simulink subsystem "s3EM"  (R2023b)
settings: Solver=VariableStepAuto  StartTime=0.0  StopTime=10.0  RelTol=1e-3
settings Model: Creator=The MathWorks, Inc.  LastModifiedBy=The MathWorks, Inc.

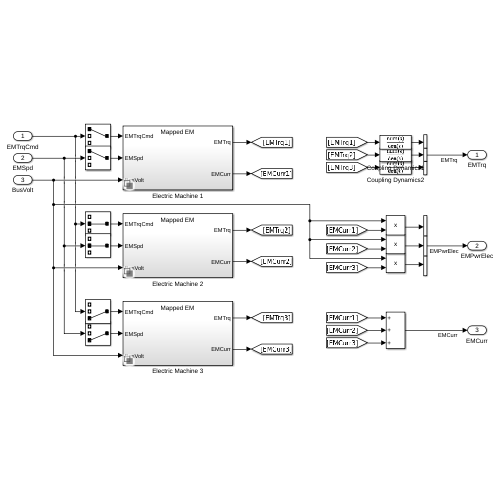
[thumbnail: Simulink's stored preview of the top-level diagram]
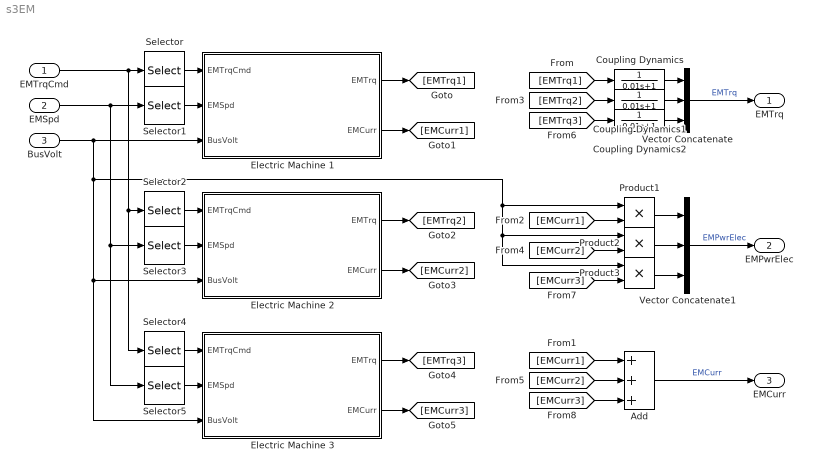
== system s3EM ==
  EMTrqCmd : Inport
  EMSpd : Inport  Port=2
  BusVolt : Inport  Port=3
  Add : Sum  Inputs=+++
  Coupling Dynamics : TransferFcn  Denominator=[0.01 1]
  Coupling Dynamics1 : TransferFcn  Denominator=[0.01 1]
  Coupling Dynamics2 : TransferFcn  Denominator=[0.01 1]
  Electric Machine 1 : Subsystem  Variant=on  VariantControlMode=label  LabelModeActiveChoice=Mapped EM
  Electric Machine 2 : Subsystem  Variant=on  VariantControlMode=label  LabelModeActiveChoice=Mapped EM
  Electric Machine 3 : Subsystem  Variant=on  VariantControlMode=label  LabelModeActiveChoice=Mapped EM
  Product1 : Product
  Product2 : Product
  Product3 : Product
  Selector : Selector  InputPortWidth=3  IndexOptions=Index vector (dialog)  Indices=[1]  OutputSizes=1
  Selector1 : Selector  InputPortWidth=3  IndexOptions=Index vector (dialog)  Indices=[1]  OutputSizes=1
  Selector2 : Selector  InputPortWidth=3  IndexOptions=Index vector (dialog)  Indices=[2]  OutputSizes=1
  Selector3 : Selector  InputPortWidth=3  IndexOptions=Index vector (dialog)  Indices=[2]  OutputSizes=1
  Selector4 : Selector  InputPortWidth=3  IndexOptions=Index vector (dialog)  Indices=[3]  OutputSizes=1
  Selector5 : Selector  InputPortWidth=3  IndexOptions=Index vector (dialog)  Indices=[3]  OutputSizes=1
  Vector Concatenate : Concatenate  NumInputs=3
  Vector Concatenate1 : Concatenate  NumInputs=3
  EMTrq : Outport
  EMPwrElec : Outport  Port=2
  EMCurr : Outport  Port=3
  wires:
  [EMTrq3] -> Coupling Dynamics2/1
  Coupling Dynamics2/1 -> Vector Concatenate/3
  Product3/1 -> Vector Concatenate1/3
  [EMCurr3] -> Product3/2
  [EMCurr3] -> Add/3
  Electric Machine 3/2(EMCurr) -> [EMCurr3]
  Electric Machine 3/1(EMTrq) -> [EMTrq3]
  Selector5/1 -> Electric Machine 3/2(EMSpd)
  Selector4/1 -> Electric Machine 3/1(EMTrqCmd)
  Vector Concatenate/1 -> EMTrq/1  "EMTrq"
  BusVolt/1 -> Electric Machine 1/3(BusVolt), Electric Machine 3/3(BusVolt), Electric Machine 2/3(BusVolt), Product1/1, Product3/1, Product2/1
  Coupling Dynamics/1 -> Vector Concatenate/1
  Vector Concatenate1/1 -> EMPwrElec/1  "EMPwrElec"
  Selector1/1 -> Electric Machine 1/2(EMSpd)
  Selector3/1 -> Electric Machine 2/2(EMSpd)
  EMTrqCmd/1 -> Selector4/1, Selector2/1, Selector/1
  Product1/1 -> Vector Concatenate1/1
  Product2/1 -> Vector Concatenate1/2
  Coupling Dynamics1/1 -> Vector Concatenate/2
  Selector2/1 -> Electric Machine 2/1(EMTrqCmd)
  Add/1 -> EMCurr/1  "EMCurr"
  Selector/1 -> Electric Machine 1/1(EMTrqCmd)
  EMSpd/1 -> Selector5/1, Selector3/1, Selector1/1
  Electric Machine 1/1(EMTrq) -> [EMTrq1]
  [EMTrq1] -> Coupling Dynamics/1
  Electric Machine 1/2(EMCurr) -> [EMCurr1]
  [EMCurr1] -> Add/1
  [EMCurr1] -> Product1/2
  [EMTrq2] -> Coupling Dynamics1/1
  [EMCurr2] -> Product2/2
  [EMCurr2] -> Add/2
  Electric Machine 2/1(EMTrq) -> [EMTrq2]
  Electric Machine 2/2(EMCurr) -> [EMCurr2]

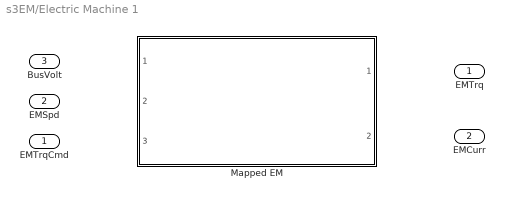
== system s3EM/Electric Machine 1 ==
  EMTrqCmd : Inport
  EMSpd : Inport  Port=2
  BusVolt : Inport  Port=3
  Mapped EM : Subsystem  VariantControl=Mapped EM  ReferencedSubsystem=ElectricMachine1
  EMTrq : Outport  VectorParamsAs1DForOutWhenUnconnected=off
  EMCurr : Outport  Port=2  VectorParamsAs1DForOutWhenUnconnected=off

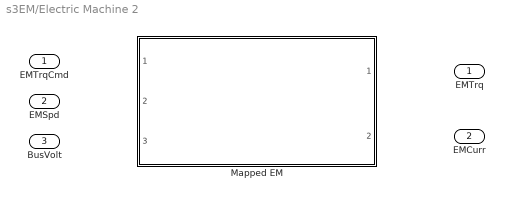
== system s3EM/Electric Machine 2 ==
  EMTrqCmd : Inport
  EMSpd : Inport  Port=2
  BusVolt : Inport  Port=3
  Mapped EM : Subsystem  VariantControl=Mapped EM  ReferencedSubsystem=ElectricMachine2
  EMTrq : Outport  VectorParamsAs1DForOutWhenUnconnected=off
  EMCurr : Outport  Port=2  VectorParamsAs1DForOutWhenUnconnected=off

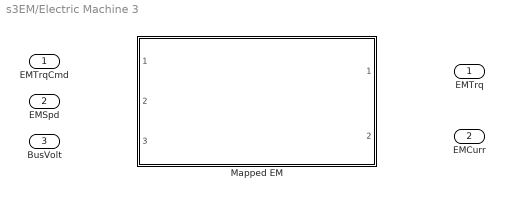
== system s3EM/Electric Machine 3 ==
  EMTrqCmd : Inport
  EMSpd : Inport  Port=2
  BusVolt : Inport  Port=3
  Mapped EM : Subsystem  VariantControl=Mapped EM  ReferencedSubsystem=ElectricMachine3
  EMTrq : Outport  VectorParamsAs1DForOutWhenUnconnected=off
  EMCurr : Outport  Port=2  VectorParamsAs1DForOutWhenUnconnected=off
